simulink model "mrand_bpsk_2u_mp"  (Simulink 6.0)
settings: Solver=ode45  StartTime=0.0  StopTime=0.125 -(1/19200)  RelTol=1e-3
libraries: mspread x8, commutil2 x2, commsink2 x2, commrandsrc2 x2, commseqgen2 x2, commchan2 x1
CloseFcn:
  | clear spreadSigsOut
settings Model: Creator=akansal  LastModifiedBy=mmclerno  ProdHWDeviceType=Specified
settings DataIOCC: SaveTime=off  SignalLoggingName=spreadSigsOut
settings OptimizationCC: BooleanDataType=off  InlineParams=on  InlineInvariantSignals=off  MultiInstanced=off
settings FormatCC: IgnoreBidirectionalLines=off
settings HardwareCC: ProdHWDeviceType=Specified
settings CodeAppCC: SimulinkBlockComments=off
settings GRTTargetCC: TargetFcnLib=iso_c_tmw.mat

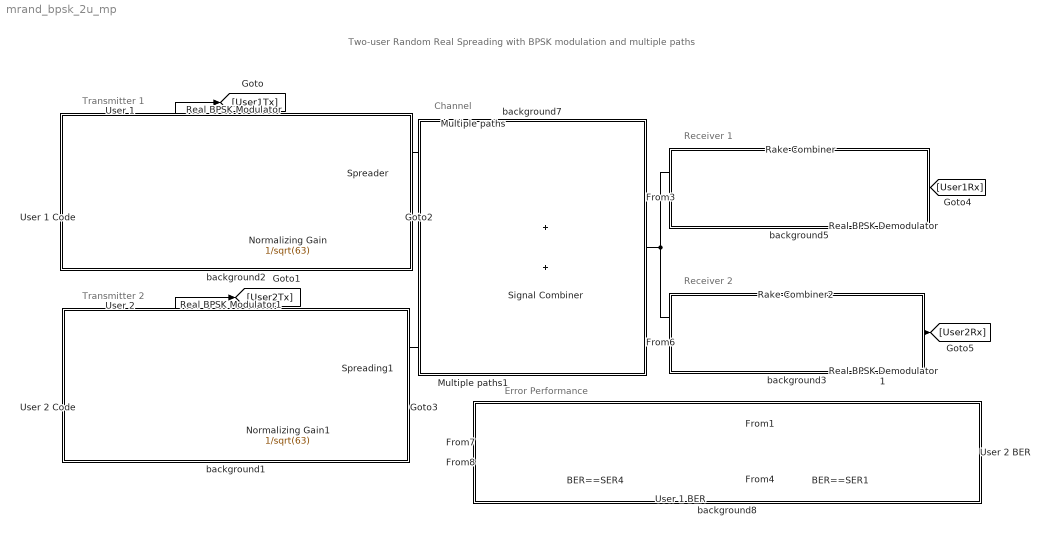
== system mrand_bpsk_2u_mp ==
  note: Two-user Random Real Spreading with BPSK modulation and multiple paths
  note: Error Performance
  note: Transmitter 1
  note: Transmitter 2
  note: Channel
  note: Receiver 1
  note: Receiver 2
  " " : commchan2/AWGN Channel  seed=1237  noiseMode="Signal to noise ratio  (SNR)"  EbNodB=10  EsNodB=25  SNRdB=5  bitsPerSym=1  Ps=1  Tsym=ts  variance=1
  "  " : commutil2/Unipolar to Bipolar Converter  M=2  polarity=Negative
  "   " : commutil2/Unipolar to Bipolar Converter  M=2  polarity=Negative
  BER==SER1 : commsink2/Error Rate Calculation  N=0  st_delay=0  cp_mode=Entire frame  subframe=[]  PMode=Port  WsName=ErrorVec  RsMode2=off  stop=off  numErr=100  maxBits=1e6
  BER==SER4 : commsink2/Error Rate Calculation  N=0  st_delay=0  cp_mode=Entire frame  subframe=[]  PMode=Port  WsName=ErrorVec  RsMode2=off  stop=off  numErr=100  maxBits=1e6
  Multiple paths : mspread/Multiple paths  p=3  pd=[0 2 6]  ts=1/19200
  Multiple paths1 : mspread/Multiple paths  p=3  pd=[0 3 5]  ts=1/19200
  Normalizing Gain : Gain  Gain=1/sqrt(63)  SaturateOnIntegerOverflow=on
  Normalizing Gain1 : Gain  Gain=1/sqrt(63)  SaturateOnIntegerOverflow=on
  Rake Combiner : mspread/Rake Combiner  pd=[0 2 6]  pgain=63
  Rake Combiner2 : mspread/Rake Combiner  pd=[0 3 5]  pgain=63
  Real BPSK Demodulator : mspread/Real BPSK Demodulator
  Real BPSK Demodulator1 : mspread/Real BPSK Demodulator
  Real BPSK Modulator : mspread/Real BPSK Modulator
  Real BPSK Modulator1 : mspread/Real BPSK Modulator
  Signal Combiner : Sum  SaturateOnIntegerOverflow=on
  Spreader : Product  SaturateOnIntegerOverflow=on  InputSameDT=on
  Spreading1 : Product  SaturateOnIntegerOverflow=on  InputSameDT=on
  User 1 : commrandsrc2/Random Integer Generator  mul=2  seed=37  Ts=1/19200  frameBased=on  sampPerFrame=1  orient=off
  "User 1 BER " : Display
  User 1 Code : Subsystem  BlockChoice=PN Sequence Generator
      link override Gold Sequence Generator: index=7  ts=1/(9600*2*63)  frameBased=on  sampPerFrame=63
      link override Kasami Sequence Generator: codeIdx=4  ts=1/(9600*2*63)  frameBased=on  sampPerFrame=63
      link override PN Sequence Generator: Ts=1/(19200*63)  frameBased=on  sampPerFrame=63
      settings: AttributesFormatString=%<BlockChoice>  TemplateBlock=randcodes/Configurable System  MemberBlocks=Gold Sequence Generator,Kasami Sequence Generator,PN Sequence Generator
  User 2 : commrandsrc2/Random Integer Generator  mul=2  seed=631  Ts=1/19200  frameBased=on  sampPerFrame=1  orient=off
  "User 2 BER " : Display
  User 2 Code : Subsystem  BlockChoice=PN Sequence Generator
      link override Gold Sequence Generator: index=2  ts=1/(9600*2*63)  frameBased=on  sampPerFrame=63
      link override Kasami Sequence Generator: genPoly=[1 1 0 1 1 0 1]  codeIdx=3  ts=1/(9600*2*63)  frameBased=on  sampPerFrame=63
      link override PN Sequence Generator: Ts=1/(19200*63)  frameBased=on  sampPerFrame=63  poly=[1 1 0 1 1 0 1]
      settings: AttributesFormatString=%<BlockChoice>  TemplateBlock=randcodes/Configurable System  MemberBlocks=Gold Sequence Generator,Kasami Sequence Generator,PN Sequence Generator
  background1 : Subsystem
      mask Display: disp('')
  background2 : Subsystem
      mask Display: disp('')
  background3 : Subsystem
      mask Display: disp('')
  background5 : Subsystem
      mask Display: disp('')
  background7 : Subsystem  Orientation=up
      mask Display: disp('')
  background8 : Subsystem
      mask Display: disp('')
  wires:
  User 1/1 -> [User1Tx], Real BPSK Modulator/1
  Spreader/1 -> Multiple paths/1
  "  "/1 -> Normalizing Gain/1
  Normalizing Gain/1 -> Spreader/2, [User1Code]
  User 2/1 -> [User2Tx], Real BPSK Modulator1/1
  Real BPSK Modulator1/1 -> Spreading1/1
  Spreading1/1 -> Multiple paths1/1
  Multiple paths/1 -> Signal Combiner/1
  Multiple paths1/1 -> Signal Combiner/2
  User 1 Code/1(Out1) -> "  "/1
  Normalizing Gain1/1 -> [User2Code], Spreading1/2
  User 2 Code/1(Out1) -> "   "/1
  "   "/1 -> Normalizing Gain1/1
  Real BPSK Modulator/1 -> Spreader/1
  " "/1 -> Rake Combiner/1, Rake Combiner2/1
  Rake Combiner/1 -> Real BPSK Demodulator/1
  [User1Code] -> Rake Combiner/2
  Rake Combiner2/1 -> Real BPSK Demodulator1/1
  [User2Code] -> Rake Combiner2/2
  [User2Tx] -> BER==SER1/1
  [User2Rx] -> BER==SER1/2
  BER==SER4/1 -> "User 1 BER "/1
  [User1Tx] -> BER==SER4/1
  [User1Rx] -> BER==SER4/2
  Real BPSK Demodulator/1 -> [User1Rx]
  Real BPSK Demodulator1/1 -> [User2Rx]
  Signal Combiner/1 -> " "/1
  BER==SER1/1 -> "User 2 BER "/1

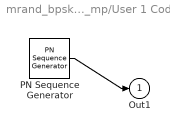
== system mrand_bpsk_2u_mp/User 1 Code ==
  PN Sequence Generator : commseqgen2/PN Sequence Generator  poly=[1 0 0 0 0 1 1]  ini_sta=[0 0 0 0 0 1]  shift=0  Ts=1/(19200*63)  frameBased=on  sampPerFrame=63  reset=off
  Out1 : Outport
  wires:
  PN Sequence Generator/1 -> Out1/1

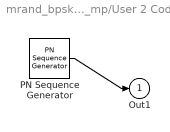
== system mrand_bpsk_2u_mp/User 2 Code ==
  PN Sequence Generator : commseqgen2/PN Sequence Generator  poly=[1 1 0 1 1 0 1]  ini_sta=[0 0 0 0 0 1]  shift=0  Ts=1/(19200*63)  frameBased=on  sampPerFrame=63  reset=off
  Out1 : Outport
  wires:
  PN Sequence Generator/1 -> Out1/1

== system mrand_bpsk_2u_mp/background1 ==

== system mrand_bpsk_2u_mp/background2 ==

== system mrand_bpsk_2u_mp/background3 ==

== system mrand_bpsk_2u_mp/background5 ==

== system mrand_bpsk_2u_mp/background7 ==

== system mrand_bpsk_2u_mp/background8 ==
